simulink model "adc_with_impairments"  (Simulink 7.4)
settings: Solver=ode45  StartTime=0.0  StopTime=10e-5  MaxStep=0.25/400e6  RelTol=1e-4
StopFcn:
  | %dt=diff(simout.time);
  | %max_step=max(dt)
  | %min_step = min(dt)
undefined symbols (not defined in the file or in its folder): One, rab_favorites, sided, Subsystem1
libraries: simulink x4, dspsnks4 x2, dspbuff3 x1, dsparch4 x1
settings Model: Creator=dbenson  LastModifiedBy=Dick
settings DataIOCC: Refine=10
settings OptimizationCC: InitFltsAndDblsToZero=on
settings DebuggingCC: SaveWithParameterizedLinksMsg=none  SignalResolutionControl=TryResolveAllWithWarning  MultiTaskDSMMsg=warning  MultiTaskCondExecSysMsg=none  StrictBusMsg=None
settings RTWCC: IncludeERTFirstTime=on
settings GRTTargetCC: TargetFcnLib=ansi_tfl_tmw.mat

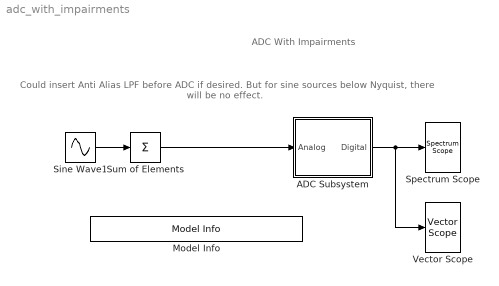
== system adc_with_impairments ==
  note: Could insert Anti Alias LPF
      | before ADC if desired. But for sine
      | sources below Nyquist, there will be no effect.
  note: ADC With Impairments
  ADC Subsystem : Subsystem
  Model Info : simulink/Model-Wide Utilities/Model Info  SystemSampleTime=-1  InitialBlockCM=None  BlockCM=None  Frame=on  DisplayStringWithTags=Copywrite 2005-2010 The MathWorks, Inc.  HorizontalTextAlignment=Center  LeftAlignmentValue=0.5  SourceBlockDiagram=adc_with_impairments  TagMaxNumber=20
  Sine Wave1 : Sin  Amplitude=.5  Bias=0  Frequency=2*pi*[20 22]*1e6  Phase=0  Samples=10  SampleTime=0  Offset=0
  Spectrum Scope : dspsnks4/Spectrum Scope  DialogController=dspdialog.SpectrumScope  DialogControllerArgs=DataTag0  SystemSampleTime=-1  ScopeProperties=on  Domain=Frequency  HorizSpan=1  UseBuffer=on  BufferSize=2048  Overlap=0  inpFftLenInherit=off  FFTlength=128  numAvg=2  DisplayProperties=off  AxisGrid=on  Memory=off  FrameNumber=on  AxisLegend=off  AxisZoom=off  OpenScopeAtSimStart=on  OpenScopeImmediately=off  FigPos=[13 485 399 237]  AxisProperties=off  XUnits=Hertz  XRange=One-sided ([0...Fs/2])  XDisplay=0  InheritXIncr=on  XIncr=1.0  XLabel=Samples  XLimit=Auto  YUnits=dBW/Hertz  XMax=1  XMin=0  YLabel=Magnitude-squared, dB  LineProperties=off  wintypeSpecScope=Hann  RsSpecScope=50  betaSpecScope=5  winsampSpecScope=Periodic  XAxisParamsVer=6.8
      settings: YMin=-146.5665  YMax=-53.7967
  Sum of Elements : Sum  Inputs=+  OutDataType=sfix(16)  OutScaling=2^-10
  Vector Scope : dspsnks4/Vector Scope  DialogController=dspdialog.VectorScope  DialogControllerArgs=DataTag1  ScopeProperties=on  Domain=Time  HorizSpan=1  DisplayProperties=off  AxisGrid=on  Memory=on  FrameNumber=on  AxisLegend=off  AxisZoom=off  OpenScopeAtSimStart=on  OpenScopeImmediately=off  FigPos=[420 485 533 238]  AxisProperties=off  XUnits=Hertz  XRange=[0...Fs/2]  InheritXIncr=on  XIncr=1  XLabel=Time  XLimit=Auto  XMin=0  XMax=1  XStart=0  YUnits=dB  YLabel=Amplitude  LineProperties=off  XAxisParamsVer=6.8
      settings: YMin=-1  YMax=1
  wires:
  Sine Wave1/1 -> Sum of Elements/1
  Sum of Elements/1 -> ADC Subsystem/1(Analog)
  ADC Subsystem/1(Digital) -> Spectrum Scope/1, Vector Scope/1

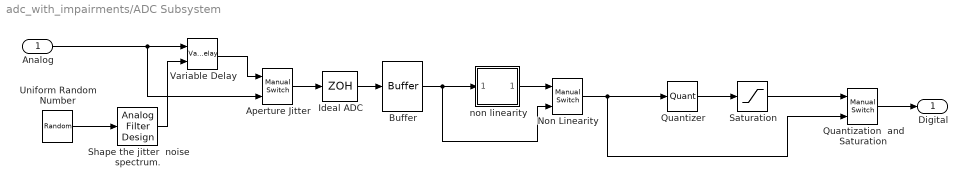
== system adc_with_impairments/ADC Subsystem ==
  Analog : Inport  OutDataType=sfix(16)  OutScaling=2^0
  Aperture Jitter : simulink/Signal Routing/Manual Switch  SystemSampleTime=-1  sw=0  action=0  varsize=off
  Buffer : dspbuff3/Buffer  N=50  V=0  ic=0
  Ideal ADC : ZeroOrderHold  SampleTime=1/100e6
  Non Linearity : simulink/Signal Routing/Manual Switch  SystemSampleTime=-1  sw=0  action=0  varsize=off
  Quantization  and Saturation : simulink/Signal Routing/Manual Switch  SystemSampleTime=-1  sw=0  action=0  varsize=off
  Quantizer : Quantizer  QuantizationInterval=2^-8
  Saturation : Saturate  UpperLimit=1  LowerLimit=-1
  "Shape the jitter  noise spectrum. " : dsparch4/Analog Filter Design  method=Butterworth  filttype=Lowpass  N=3  Wlo=2*pi*4e6  Whi=80  Rp=2  Rs=40
  Uniform Random Number : UniformRandomNumber  Minimum=0  Maximum=5e-9  Seed=1234  SampleTime="0 %  1/100e6"
  Variable Delay : VariableTransportDelay  MaximumDelay=30e-9  ZeroDelay=on  TransDelayFeedthrough=on
  non linearity : Subsystem  AncestorBlock=rab_favorites/Subsystem1  mask{alpha=.2}
      mask init:
      | x=-3:0.01:3;  y= (1/alpha)*tanh(alpha*x) ;
      mask Display: plot(x,y)
  Digital : Outport  OutDataType=sfix(16)  OutScaling=2^0
  wires:
  Uniform Random Number/1 -> "Shape the jitter  noise spectrum. "/1
  Quantizer/1 -> Saturation/1
  Aperture Jitter/1 -> Ideal ADC/1
  Variable Delay/1 -> Aperture Jitter/1
  Saturation/1 -> Quantization  and Saturation/1
  "Shape the jitter  noise spectrum. "/1 -> Variable Delay/2
  Ideal ADC/1 -> Buffer/1
  non linearity/1(Out1) -> Non Linearity/1
  Non Linearity/1 -> Quantizer/1, Quantization  and Saturation/2
  Analog/1 -> Aperture Jitter/2, Variable Delay/1
  Buffer/1 -> non linearity/1(In1), Non Linearity/2
  Quantization  and Saturation/1 -> Digital/1

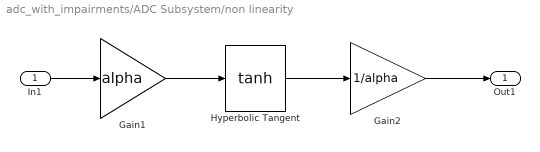
== system adc_with_impairments/ADC Subsystem/non linearity ==
  In1 : Inport  OutDataType=sfix(16)  OutScaling=2^0
  Gain1 : Gain  Gain=alpha  ParameterDataType=sfix(16)  ParameterScaling=2^0  OutDataType=sfix(16)  OutScaling=2^0  SaturateOnIntegerOverflow=on  OutDataTypeStr=Inherit: Same as input  ParamDataTypeStr=Inherit: Same as input
  Gain2 : Gain  Gain=1/alpha  ParameterDataType=sfix(16)  ParameterScaling=2^0  OutDataType=sfix(16)  OutScaling=2^0  SaturateOnIntegerOverflow=on  OutDataTypeStr=Inherit: Same as input  ParamDataTypeStr=Inherit: Same as input
  Hyperbolic Tangent : Trigonometry  Operator=tanh
  Out1 : Outport  OutDataType=sfix(16)  OutScaling=2^0
  wires:
  Hyperbolic Tangent/1 -> Gain2/1
  In1/1 -> Gain1/1
  Gain2/1 -> Out1/1
  Gain1/1 -> Hyperbolic Tangent/1
